simulink model "RT_sys_2nd_order"  (Simulink 8.1)
settings: Solver=ode45  StartTime=0.0  StopTime=1  RelTol=1e-3
values from neighbouring files (symbols this model uses):
  a = [2 3 5 8]    [RT_lab_paramLead.m]    (also in RT_lead_lag_uebung.m = aa(i); RT_sys_2nd_order_post.m = 0.1)
  b = [-2;1]    [RT_dennis_draussen.m]    (also in RT_klausurvorb.m = [1;0]; RT_sys_2nd_order_post.m = 5; RT_ueb2_proc.m = [0;3]; sys2order_post.m = [0;1/(J*R)])
libraries: simulink x1
settings Model: Creator=mainster  LastModifiedBy=mainster
settings SolverCC: MaxConsecutiveMinStep=5

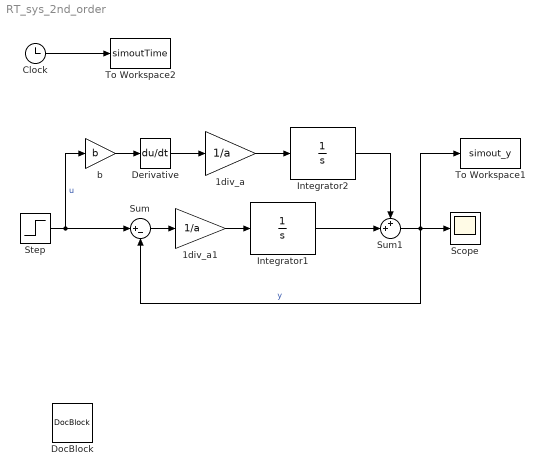
== system RT_sys_2nd_order ==
  1div_a : Gain  Gain=1/a
  1div_a1 : Gain  Gain=1/a
  Clock : Clock
  Derivative : Derivative
  DocBlock : simulink/Model-Wide Utilities/DocBlock  DocumentType=Text
  Integrator1 : Integrator  UpperSaturationLimit=1e6  LowerSaturationLimit=-1e5
  Integrator2 : Integrator  UpperSaturationLimit=1e6  LowerSaturationLimit=-1e5
  Scope : Scope
  Step : Step  Time=10e-3  SampleTime=0
  Sum : Sum  Inputs=|+-
  Sum1 : Sum  Inputs=++|
  To Workspace1 : ToWorkspace  VariableName=simout_y  SampleTime=-1  SaveFormat=Structure
  To Workspace2 : ToWorkspace  VariableName=simoutTime  SampleTime=-1  SaveFormat=Structure
  b : Gain  Gain=b
  wires:
  Clock/1 -> To Workspace2/1
  Step/1 -> Sum/1, b/1  "u"
  Sum/1 -> 1div_a1/1
  1div_a1/1 -> Integrator1/1
  Integrator1/1 -> Sum1/2
  1div_a/1 -> Integrator2/1
  Integrator2/1 -> Sum1/1
  b/1 -> Derivative/1
  Derivative/1 -> 1div_a/1
  Sum1/1 -> Scope/1, Sum/2, To Workspace1/1  "y"
